simulink model "model2_linresp"  (R2021b)
settings: Solver=VariableStepAuto  StartTime=0.0  StopTime=30  RelTol=1e-3
undefined symbols (not defined in the file or in its folder): A_lin, B_lin, C_lin, D_lin, ustarr, xstarr, ystarr
settings Model: Creator=AMY  LastModifiedBy=AMY

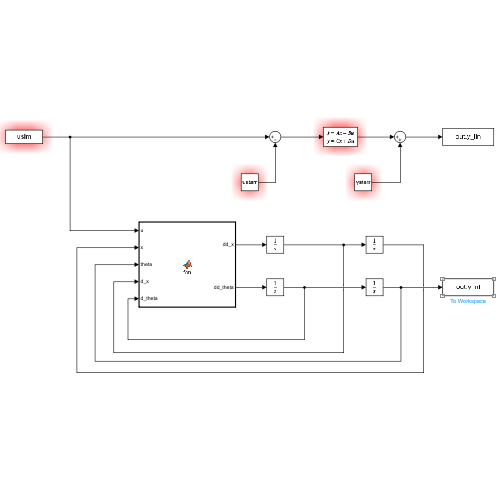
[thumbnail: Simulink's stored preview of the top-level diagram]
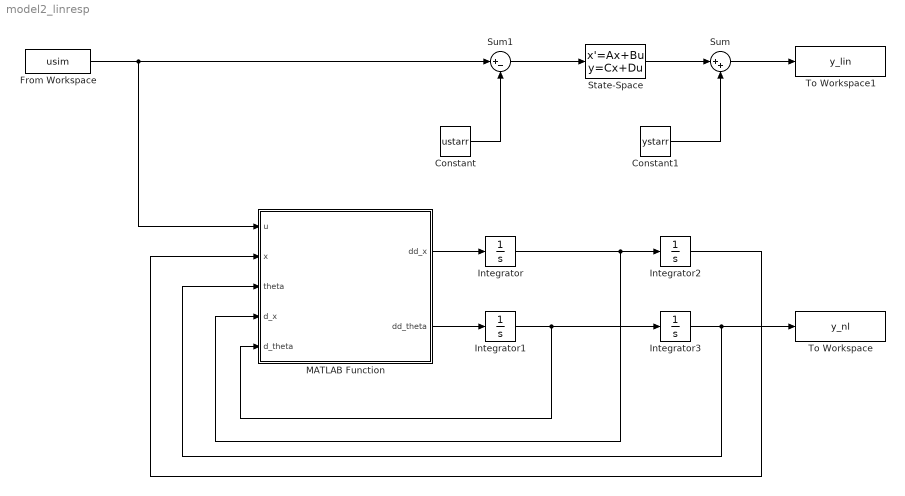
== system model2_linresp ==
  Constant : Constant  Value=ustarr
  Constant1 : Constant  Value=ystarr
  From Workspace : FromWorkspace  VariableName=usim
  Integrator{,1..3} (4 alike) : Integrator
  MATLAB Function : MATLAB Function  TreatAsAtomicUnit=on
  State-Space : StateSpace  A=A_lin  B=B_lin  C=C_lin  D=D_lin  InitialCondition=-xstarr
  Sum : Sum  Inputs=|++
  Sum1 : Sum  Inputs=|+-
  To Workspace : ToWorkspace  VariableName=y_nl  SaveFormat=Timeseries  SampleTime=-1
      settings: Save2DSignal=2-D array (concatenate along first dimension)
  To Workspace1 : ToWorkspace  VariableName=y_lin  SaveFormat=Timeseries  SampleTime=-1
  wires:
  MATLAB Function/2(dd_theta) -> Integrator1/1
  Integrator/1 -> MATLAB Function/4(d_x), Integrator2/1
  Integrator3/1 -> To Workspace/1, MATLAB Function/3(theta)
  From Workspace/1 -> Sum1/1, MATLAB Function/1(u)
  Integrator1/1 -> Integrator3/1, MATLAB Function/5(d_theta)
  Integrator2/1 -> MATLAB Function/2(x)
  MATLAB Function/1(dd_x) -> Integrator/1
  Sum1/1 -> State-Space/1
  State-Space/1 -> Sum/1
  Constant/1 -> Sum1/2
  Constant1/1 -> Sum/2
  Sum/1 -> To Workspace1/1

== matlab function model2_linresp/MATLAB Function ==
  data: dd_x output; u input; dd_theta output; x input; theta input; d_x input; d_theta input
function [dd_x, dd_theta] = fcn(u, x, theta,  d_x, d_theta)

    m = 1.5;          %Masa corpului
    g = 9.81;         %Acceleratia gravitationala
    zeta = 0.6;      %Coeficient de amortizare
    k = 1.5;          %Constanta elastica
    l0 = 0.5;         %Lungimea initiala a resortului
    
    %Ecuatiile
    dd_x = (l0+x)*(d_theta)*(d_theta) - (k/m)*x + g*cos(theta) - zeta*d_x;
    dd_theta = -(g/(l0+x)*sin(theta))-(2*d_x/(l0+x))*d_theta - zeta*d_theta + 1/(m*(l0+x)*(l0+x))*u;

end
